simulink model "cukModelStateSpaceWithcontrol"  (R2020a)
settings: Solver=VariableStepAuto  StartTime=0.0  StopTime=0.3  RelTol=1e-9  AbsTol=4e-3
undefined symbols (not defined in the file): Asigma, b1, b2, bsigma, Csigma, Cxe, delta, f_s, fbounds, jthVec, Masigma, Mbsigma, Mcsigma, Nasigma, Nbsigma, Ncsigma, obsControl, obsSys, P, t_f, taua1, taua2, Tmax, uncertFreq, uncertType, x0, x_e, xe, xfdio0, xhat0
libraries: PhdLibrary x23, dspsigops x7, powerlib_meascontrol x5, dspmathops x1
(part 1 of 2)
settings Model: SimulationMode=accelerator  Creator=d13go  LastModifiedBy=d13go
settings SolverCC: ZeroCrossControl=DisableAll  ZeroCrossAlgorithm=Adaptive
settings DebuggingCC: IgnoredZcDiagnostic=none

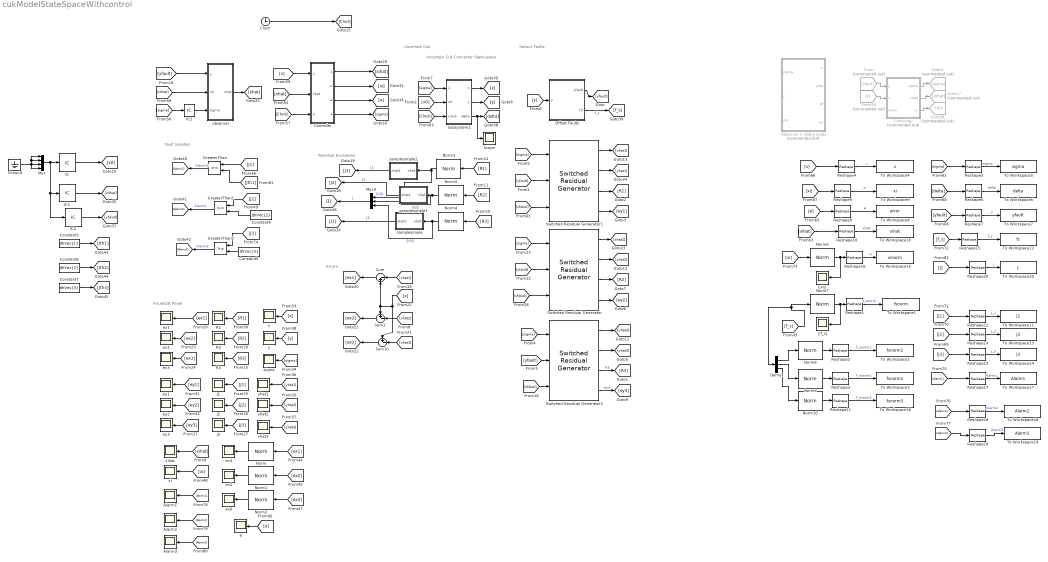
== system cukModelStateSpaceWithcontrol ==
  note: Errors
  note: Fault Isolation
  note: Visualizat Panel
  note: Sensor Faults
  note: Uncertain Cuk Converter
      | State-space
  note: Uncertain Cuk
  note: Residual Evaluation
  Alarm1 : Scope
  Alarm2 : Scope
  Alarm3 : Scope
  Clock : Clock
  Constant3 : Constant  Value=jthVec{1}
  Constant4 : Constant  Value=jthVec{2}
  Constant5 : Constant  Value=jthVec{3}
  Constant6 : Constant  Value=jthVec{2}
  Constant7 : Constant  Value=jthVec{3}
  Controler : Subsystem
  Controller : Subsystem  Commented=on
  Demux : Demux  Outputs=3
  From : From  Commented=on  GotoTag=yfault
  From50 : From  Commented=on  GotoTag=x
  Goto17 : Goto  Commented=on  GotoTag=xihat
  Goto28 : Goto  Commented=on  GotoTag=xi
  Goto4 : Goto  Commented=on  GotoTag=sigma
  GreaterThan : RelationalOperator  OutDataTypeStr=boolean  RndMeth=Simplest
  GreaterThan1 : RelationalOperator  OutDataTypeStr=boolean  RndMeth=Simplest
  GreaterThan2 : RelationalOperator  OutDataTypeStr=boolean  RndMeth=Simplest
  Ground : Ground
  IC : InitialCondition  Value=[x0]
  IC1 : InitialCondition  Value=[xhat0]
  IC2 : InitialCondition  Value=2
  IC4 : InitialCondition  Value=[xfdio0]
  J1 : Scope
  J2 : Scope
  J3 : Scope
  Mux : Mux
  Mux4 : Mux  Inputs=3
  Norm{,1..10} (11 alike) : PhdLibrary/Norms/Norm
      settings: SourceProductName=Phd Diego
  Observer 2 slidng mode : Subsystem  Commented=on  mask(Boots State-Space model){A1=obsSys{3}.Asigma{1,1}, A2=obsSys{3}.Asigma{1,2}, B1=obsSys{3}.bsigma{1,1}, Cmatrix=obsSys{3}.Csigma{1,1}, L1=obsSys{3}.Lsigma{1,1}, L2=obsSys{3}.Lsigma{1,2}, Gn1=obsSys{3}.Gnsigma{1,1}, Gn2=obsSys{3}.Gnsigma{1,2}, Po=obsSys{3}.Po, R1=obsSys{3}.Rsigma{1,1}, R2=obsSys{3}.Rsigma{1,2}, delta=delta}
      mask prompts: A1 "A1 matrix"; A2 "A2 matrix"; B1 "B matrix"; Cmatrix "Output Matrix"; L1 "L1 matrix"; L2 "L2 matrix"; Gn1 "Gn1 matrix"; Gn2 "Gn2 matrix"; Po "Po matrix"; R1 "R1 matrix"; R2 "R2 matrix"; delta "Delta Sliding mode"
      mask help: Boots State-Space model
      mask Display: disp('Observer')
  Offset Faults : Subsystem
  R1 : Scope
  R2 : Scope
  R3 : Scope
  Reshape{1..20} (20 alike) : Reshape
  Scope : Scope
  Subsystem2 : Subsystem
  Sum : Sum  Inputs=|-+
  Sum1 : Sum  Inputs=+-|
  Sum10 : Sum  Inputs=+-|
  Switched Residual Generator : PhdLibrary/Observers/Switched Residual Generator  A1=obsSys{2}.Asigma{1,1}  B1=obsSys{2}.bsigma{1,1}  L1=obsSys{2}.Lsigma{1,1}  C1=obsSys{2}.Csigma{1,1}  R1=obsSys{2}.Rsigma{1,1}  A2=obsSys{2}.Asigma{1,2}  B2=obsSys{2}.bsigma{1,1}  C2=obsSys{2}.Csigma{1,1}  L2=obsSys{2}.Lsigma{1,2}  R2=obsSys{2}.Rsigma{1,2}
      settings: SourceProductName=Phd Diego
  Switched Residual Generator1 : PhdLibrary/Observers/Switched Residual Generator  A1=obsSys{1}.Asigma{1,1}  B1=obsSys{1}.bsigma{1,1}  L1=obsSys{1}.Lsigma{1,1}  C1=obsSys{1}.Csigma{1,1}  R1=obsSys{1}.Rsigma{1,1}  A2=obsSys{1}.Asigma{1,2}  B2=obsSys{1}.bsigma{1,1}  C2=obsSys{1}.Csigma{1,1}  L2=obsSys{1}.Lsigma{1,2}  R2=obsSys{1}.Rsigma{1,2}
      settings: SourceProductName=Phd Diego
  Switched Residual Generator2 : PhdLibrary/Observers/Switched Residual Generator  A1=obsSys{3}.Asigma{1,1}  B1=obsSys{3}.bsigma{1,1}  L1=obsSys{3}.Lsigma{1,1}  C1=obsSys{3}.Csigma{1,1}  R1=obsSys{3}.Rsigma{1,1}  A2=obsSys{3}.Asigma{1,2}  B2=obsSys{3}.bsigma{1,1}  C2=obsSys{3}.Csigma{1,1}  L2=obsSys{3}.Lsigma{1,2}  R2=obsSys{3}.Rsigma{1,2}
      settings: SourceProductName=Phd Diego
  To Workspace1 : ToWorkspace  VariableName=fsnorm  SaveFormat=Timeseries  SampleTime=-1
  To Workspace10 : ToWorkspace  VariableName=xihat  SaveFormat=Timeseries  SampleTime=-1
  To Workspace11 : ToWorkspace  VariableName=J1  SaveFormat=Timeseries  SampleTime=-1
  To Workspace12 : ToWorkspace  VariableName=fs  SaveFormat=Timeseries  SampleTime=-1
  To Workspace13 : ToWorkspace  VariableName=J2  SaveFormat=Timeseries  SampleTime=-1
  To Workspace14 : ToWorkspace  VariableName=J3  SaveFormat=Timeseries  SampleTime=-1
  To Workspace15 : ToWorkspace  VariableName=xinorm  SaveFormat=Timeseries  SampleTime=-1
  To Workspace16 : ToWorkspace  VariableName=fsnorm3  SaveFormat=Timeseries  SampleTime=-1
  To Workspace17 : ToWorkspace  VariableName=Alarm1  SaveFormat=Timeseries  SampleTime=-1
  To Workspace18 : ToWorkspace  VariableName=Alarm2  SaveFormat=Timeseries  SampleTime=-1
  To Workspace19 : ToWorkspace  VariableName=Alarm3  SaveFormat=Timeseries  SampleTime=-1
  To Workspace2 : ToWorkspace  VariableName=fsnorm1  SaveFormat=Timeseries  SampleTime=-1
  To Workspace20 : ToWorkspace  VariableName=J  SaveFormat=Timeseries  SampleTime=-1
  To Workspace3 : ToWorkspace  VariableName=fsnorm2  SaveFormat=Timeseries  SampleTime=-1
  To Workspace4 : ToWorkspace  VariableName=x  SaveFormat=Timeseries  SampleTime=-1
  To Workspace5 : ToWorkspace  VariableName=sigma  SaveFormat=Timeseries  SampleTime=-1
  To Workspace6 : ToWorkspace  VariableName=delta  SaveFormat=Timeseries  SampleTime=-1
  To Workspace7 : ToWorkspace  VariableName=yfault  SaveFormat=Timeseries  SampleTime=-1
  To Workspace8 : ToWorkspace  VariableName=error  SaveFormat=Timeseries  SampleTime=-1
  To Workspace9 : ToWorkspace  VariableName=xi  SaveFormat=Timeseries  SampleTime=-1
  e : Scope
  ex{1..6} (6 alike) : Scope
  ey1 : Scope
  ey2 : Scope
  ey3 : Scope
  observer : Subsystem
  samplesimple : Subsystem
  samplesimple1 : Subsystem
  samplesimple2 : Subsystem
  sigma : Scope
  x : Scope
  xi : Scope
  xihat : Scope
  y : Scope
  yhat1 : Scope
  yhat2 : Scope
  yhat3 : Scope
  ||f_s| : Scope
  ||xi|| : Scope
  wires:
  Subsystem2/1(x) -> [x]
  Clock/1 -> [Clock]
  [sigma] -> Switched Residual Generator1/1
  Switched Residual Generator1/3 -> [R1]
  [sigma] -> Switched Residual Generator/1
  [yfault] -> Switched Residual Generator/2
  Switched Residual Generator1/4 -> [ey1]
  [yfault] -> Switched Residual Generator2/2
  [sigma] -> Switched Residual Generator2/1
  Switched Residual Generator2/2 -> [yhat3]
  Subsystem2/2(y) -> [y]
  Switched Residual Generator2/1 -> [xhat3]
  [xhat3] -> Sum10/2
  [yfault] -> Switched Residual Generator1/2
  [y] -> Offset Faults/1(y)
  Offset Faults/1(yfault) -> [yfault]
  Controller/1(sigma) -> Goto4/1
  From/1 -> Controller/1(y)
  [sigma] -> Subsystem2/1(sigma)
  [xhat2] -> Sum1/2
  Mux/1 -> IC1/1, IC4/1, IC/1
  Switched Residual Generator2/4 -> [ey3]  "ey3"
  Switched Residual Generator1/1 -> [xhat1]
  Switched Residual Generator2/3 -> [R3]  "R3"
  IC/1 -> [x0]
  [xfdio0] -> Switched Residual Generator2/3
  Ground/1 -> Mux/4, Mux/1, Mux/2, Mux/3
  [R3] -> Norm4/1
  Norm4/1 -> Mux4/3, samplesimple/1(xhat)  "||r3||"
  Norm5/1 -> samplesimple1/1(xhat), Mux4/2  "||r2||"
  [R2] -> Norm5/1
  Norm3/1 -> samplesimple2/1(xhat), Mux4/1  "||r1||"
  [R1] -> Norm3/1
  [R3] -> R3/1
  [ey3] -> ey3/1
  [xhat1] -> Sum/1
  [x] -> Sum/2, Sum1/1, Sum10/1
  Sum/1 -> [ex1]
  Sum10/1 -> [ex3]
  Sum1/1 -> [ex2]
  [ex1] -> ex1/1
  [ex2] -> ex2/1
  [ex3] -> ex3/1
  [J1] -> J1/1
  [J3] -> J3/1
  [J2] -> J2/1
  [xfdio0] -> Switched Residual Generator/3
  Switched Residual Generator/3 -> [R2]
  Switched Residual Generator/4 -> [ey2]
  Switched Residual Generator/2 -> [yhat2]
  Switched Residual Generator/1 -> [xhat2]
  [xfdio0] -> Switched Residual Generator1/3
  Switched Residual Generator1/2 -> [yhat1]
  [R2] -> R2/1
  [R1] -> R1/1
  [ey1] -> ey1/1
  [ey2] -> ey2/1
  [x] -> x/1
  [sigma] -> sigma/1
  [yhat2] -> yhat2/1
  [yhat1] -> yhat1/1
  [yhat3] -> yhat3/1
  [y] -> y/1
  [ex1] -> Norm/1
  Norm/1 -> ex4/1
  Norm1/1 -> ex5/1
  [ex2] -> Norm1/1
  Norm2/1 -> ex6/1
  [ex3] -> Norm2/1
  Controller/2(xihat) -> Goto17/1
  Controller/3(xi) -> Goto28/1
  [xihat] -> xihat/1
  [xi] -> xi/1
  From50/1 -> Controller/2(x)
  IC2/1 -> observer/3(sigma)
  [xhat] -> Controler/2(xhat)
  observer/1(xhat) -> [xhat]
  [x] -> Controler/1(x)
  [sigma] -> IC2/1
  [Clock] -> Controler/3(clock)
  Controler/4(sigma) -> [sigma]
  Controler/3(e) -> [e]
  Controler/2(xi) -> [xi]
  Controler/1(xihat) -> [xihat]
  [yfault] -> observer/1(y)
  [x0hat] -> observer/2(x0)
  IC1/1 -> [x0hat]
  [e] -> e/1
  IC4/1 -> [xfdio0]
  [x0] -> Subsystem2/2(x0)
  [e] -> Reshape8/1
  Reshape4/1 -> To Workspace4/1  "x"
  Reshape8/1 -> To Workspace8/1  "e"
  [delta] -> Reshape6/1
  Reshape5/1 -> To Workspace5/1  "sigma"
  Reshape7/1 -> To Workspace7/1  "y"
  Reshape6/1 -> To Workspace6/1  "delta"
  [yfault] -> Reshape7/1
  [sigma] -> Reshape5/1
  [x] -> Reshape4/1
  [xi] -> Reshape9/1
  Reshape9/1 -> To Workspace9/1  "xi"
  Reshape10/1 -> To Workspace10/1  "xihat"
  [xihat] -> Reshape10/1
  Reshape12/1 -> To Workspace11/1  "J_1"
  [J1] -> Reshape12/1
  Reshape13/1 -> To Workspace14/1  "J_3"
  Reshape14/1 -> To Workspace13/1  "J_2"
  [J2] -> Reshape14/1
  [J3] -> Reshape13/1
  Offset Faults/2(f3) -> [f_s]  "f_s"
  Reshape15/1 -> To Workspace12/1  "f_s"
  [f_s] -> Reshape15/1
  Reshape16/1 -> To Workspace15/1  "xi"
  [xi] -> Norm6/1
  Norm6/1 -> ||xi||/1, Reshape16/1
  Norm7/1 -> ||f_s|/1, Reshape1/1
  Reshape1/1 -> To Workspace1/1  "f_snorm"
  [f_s] -> Norm7/1, Demux/1
  Reshape2/1 -> To Workspace2/1  "f_snorm1"
  Demux/1 -> Norm8/1
  Norm8/1 -> Reshape2/1
  Norm9/1 -> Reshape3/1
  Reshape3/1 -> To Workspace3/1  "f_snorm2"
  Demux/2 -> Norm9/1
  Reshape11/1 -> To Workspace16/1  "f_snorm3"
  Demux/3 -> Norm10/1
  Norm10/1 -> Reshape11/1
  [J1] -> GreaterThan/1
  [Jth1] -> GreaterThan/2
  Constant5/1 -> GreaterThan2/2
  [J3] -> GreaterThan2/1
  [J2] -> GreaterThan1/1
  Constant4/1 -> GreaterThan1/2
  GreaterThan/1 -> [Alarm1]  "Alarrm1"
  GreaterThan2/1 -> [Alarm3]  "Alarm3"
  GreaterThan1/1 -> [Alarm2]  "Alarm2"
  Reshape17/1 -> To Workspace17/1  "Alarm1"
  [Alarm1] -> Reshape17/1
  [Alarm2] -> Reshape18/1
  Reshape18/1 -> To Workspace18/1  "Alarm2"
  [Alarm3] -> Reshape19/1
  Reshape19/1 -> To Workspace19/1  "Alarm3"
  [Alarm1] -> Alarm1/1
  [Alarm2] -> Alarm2/1
  [Alarm3] -> Alarm3/1
  Constant3/1 -> [Jth1]
  Constant6/1 -> [Jth2]
  Constant7/1 -> [Jth3]
  Reshape20/1 -> To Workspace20/1  "J"
  [J] -> Reshape20/1
  [Clock] -> Subsystem2/3(clock)
  samplesimple1/1("xhatk ") -> [J2]  "J2"
  samplesimple2/1("xhatk ") -> [J1]  "J1"
  Mux4/1 -> [J]  "J"
  samplesimple/1("xhatk ") -> [J3]  "J3"
  Subsystem2/3(delta) -> Scope/1, [delta]

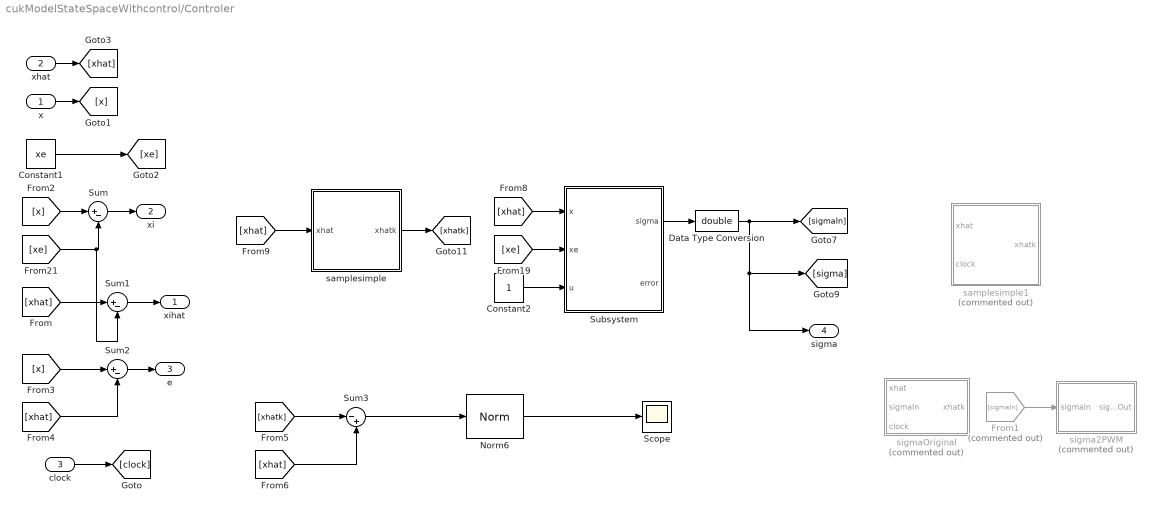
== system cukModelStateSpaceWithcontrol/Controler ==
  x : Inport
  xhat : Inport  Port=2
  clock : Inport  Port=3
  Constant1 : Constant  Value=xe  VectorParams1D=off
  Constant2 : Constant
  Data Type Conversion : DataTypeConversion  OutDataTypeStr=double
  From1 : From  Commented=on  GotoTag=sigmaIn
  Norm6 : PhdLibrary/Norms/Norm
      settings: SourceProductName=Phd Diego
  Scope : Scope
  Subsystem : Subsystem  mask{P1=P, A1=obsControl.Asigma{1}, B1=obsControl.bsigma{1}, P2=P, A2=obsControl.Asigma{2}, B2=obsControl.bsigma{2}}
      mask prompts: P1 "P matrx"; A1 "A matrix"; B1 "b matrix"; P2 "P matrx"; A2 "A matrix"; B2 "b matrix"
      mask DialogControl Container3 Prompt: Subsystem 1
      mask DialogControl Container3_copy Prompt: Subsystem 2
      mask Display: disp('Switching \n Control Law \n 2-Subsystems');
  Sum : Sum  Inputs=|+-
  Sum1 : Sum  Inputs=|+-
  Sum2 : Sum  Inputs=|+-
  Sum3 : Sum  Inputs=|-+
  samplesimple : Subsystem
  samplesimple1 : Subsystem  Commented=on
  sigma2PWM : Subsystem  Commented=on
  sigmaOriginal : Subsystem  Commented=on
  xihat : Outport
  xi : Outport  Port=2
  e : Outport  Port=3
  sigma : Outport  Port=4
  wires:
  [xe] -> Sum1/2, Sum/2
  xhat/1 -> [xhat]
  x/1 -> [x]
  Sum2/1 -> e/1
  samplesimple/1("xhatk ") -> [xhatk]
  Sum1/1 -> xihat/1
  [xe] -> Subsystem/2(xe)
  Constant2/1 -> Subsystem/3(u)
  Subsystem/1(sigma) -> Data Type Conversion/1
  Data Type Conversion/1 -> sigma/1, [sigma], [sigmaIn]
  From1/1 -> sigma2PWM/1(sigmaIn)
  clock/1 -> [clock]
  Sum/1 -> xi/1
  Constant1/1 -> [xe]
  [xhat] -> Sum1/1
  [x] -> Sum/1
  [x] -> Sum2/1
  [xhat] -> Sum2/2
  [xhatk] -> Sum3/1
  Sum3/1 -> Norm6/1
  [xhat] -> Sum3/2
  Norm6/1 -> Scope/1
  [xhat] -> samplesimple/1(xhat)
  [xhat] -> Subsystem/1(x)

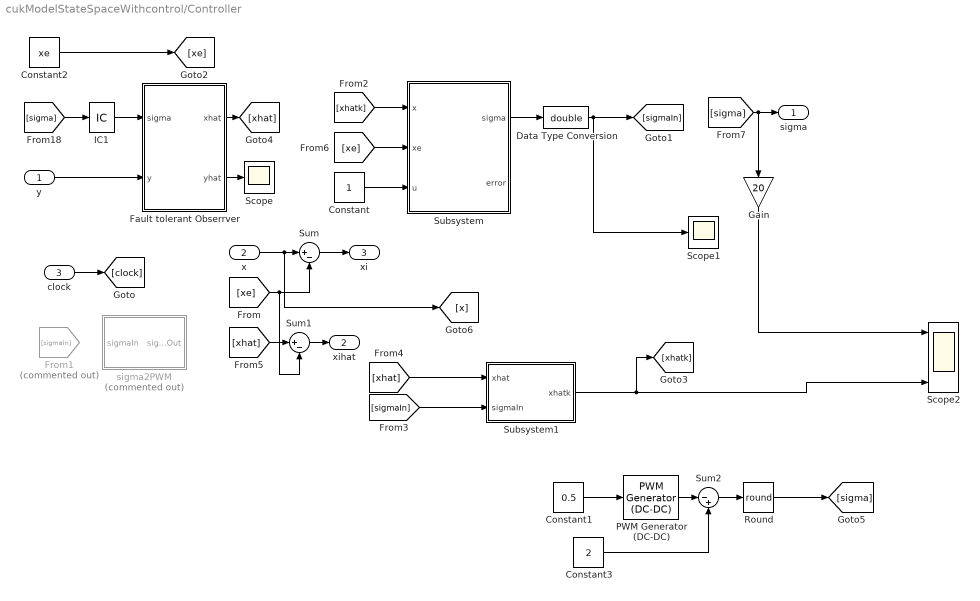
== system cukModelStateSpaceWithcontrol/Controller ==
  y : Inport
  x : Inport  Port=2
  clock : Inport  Port=3
  Constant : Constant
  Constant1 : Constant  Value=0.5
  Constant2 : Constant  Value=xe  VectorParams1D=off
  Constant3 : Constant  Value=2
  Data Type Conversion : DataTypeConversion  OutDataTypeStr=double
  Fault tolerant Obserrver : Subsystem  mask(Boots State-Space model){A1=obsControl.Asigma{1,1}, A2=obsControl.Asigma{1,2}, B1=obsControl.bsigma{1,1}, Cmatrix=obsControl.Csigma{1,1}, L1=obsControl.Lcsigma{1,1}, L2=obsControl.Lcsigma{1,2}}
      mask prompts: A1 "A1 matrix"; A2 "A2 matrix"; B1 "B matrix"; Cmatrix "Output Matrix"; L1 "L1 matrix"; L2 "L2 matrix"
      mask help: Boots State-Space model
      mask Display: disp('Observer')
  From1 : From  Commented=on  GotoTag=sigmaIn
  Gain : Gain  Gain=20
  IC1 : InitialCondition  Value=2
  PWM Generator (DC-DC) : powerlib_meascontrol/Pulse & Signal Generators/PWM Generator (DC-DC)  Fsw=10000  Ts=5e-6
  Round : Rounding  Operator=round
  Scope : Scope
  Scope1 : Scope
  Scope2 : Scope  NumInputPorts=3
  Subsystem : Subsystem  mask{P1=obsControl.P{1}, A1=obsControl.Asigma{1}, B1=obsControl.bsigma{1}, P2=obsControl.P{2}, A2=obsControl.Asigma{2}, B2=obsControl.bsigma{2}}
      mask prompts: P1 "P matrx"; A1 "A matrix"; B1 "b matrix"; P2 "P matrx"; A2 "A matrix"; B2 "b matrix"
      mask DialogControl Container3 Prompt: Subsystem 1
      mask DialogControl Container3_copy Prompt: Subsystem 2
      mask Display: disp('Switching \n Control Law \n 2-Subsystems');
  Subsystem1 : Subsystem
  Sum : Sum  Inputs=|+-
  Sum1 : Sum  Inputs=|+-
  Sum2 : Sum  Inputs=|-+
  sigma2PWM : Subsystem  Commented=on
  sigma : Outport
  xihat : Outport  Port=2
  xi : Outport  Port=3
  wires:
  [sigma] -> IC1/1
  Fault tolerant Obserrver/2(yhat) -> Scope/1
  y/1 -> Fault tolerant Obserrver/2(y)
  Fault tolerant Obserrver/1(xhat) -> [xhat]
  Constant2/1 -> [xe]
  IC1/1 -> Fault tolerant Obserrver/1(sigma)
  Constant/1 -> Subsystem/3(u)
  x/1 -> [x], Sum/1
  [xe] -> Sum/2, Sum1/2
  Sum/1 -> xi/1
  clock/1 -> [clock]
  Subsystem/1(sigma) -> Data Type Conversion/1
  Data Type Conversion/1 -> Scope1/1, [sigmaIn]
  [sigma] -> Gain/1, sigma/1
  Gain/1 -> Scope2/1
  Subsystem1/1("xhatk ") -> [xhatk], Scope2/3
  [sigmaIn] -> Subsystem1/2(sigmaIn)
  [xhat] -> Sum1/1
  Sum1/1 -> xihat/1
  [xe] -> Subsystem/2(xe)
  [xhat] -> Subsystem1/1(xhat)
  [xhatk] -> Subsystem/1(x)
  Constant1/1 -> PWM Generator (DC-DC)/1
  Constant3/1 -> Sum2/2
  Sum2/1 -> Round/1
  PWM Generator (DC-DC)/1 -> Sum2/1
  Round/1 -> [sigma]

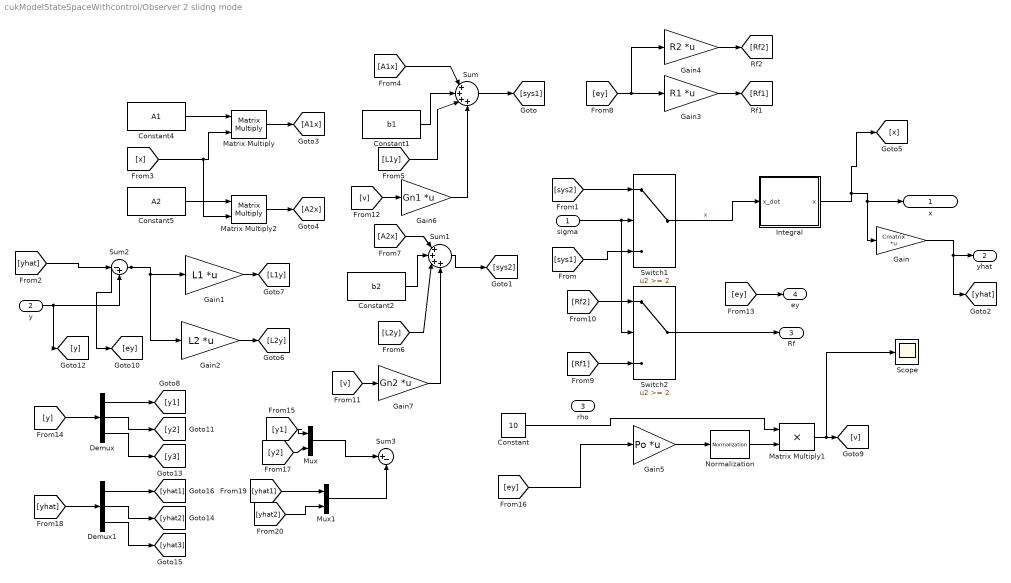
== system cukModelStateSpaceWithcontrol/Observer 2 slidng mode ==
  sigma : Inport
  y : Inport  Port=2
  rho : Inport  Port=3
  Constant : Constant  Value=10
  Constant1 : Constant  Value=b1  VectorParams1D=off
  Constant2 : Constant  Value=b2  VectorParams1D=off
  Constant4 : Constant  Value=A1  VectorParams1D=off
  Constant5 : Constant  Value=A2  VectorParams1D=off
  Demux : Demux  Outputs=3
  Demux1 : Demux  Outputs=3
  Gain : Gain  Gain=Cmatrix  Multiplication=Matrix(K*u)
  Gain1 : Gain  Gain=L1  Multiplication=Matrix(K*u) (u vector)
  Gain2 : Gain  Gain=L2  Multiplication=Matrix(K*u) (u vector)
  Gain3 : Gain  Gain=R1  Multiplication=Matrix(K*u) (u vector)
  Gain4 : Gain  Gain=R2  Multiplication=Matrix(K*u) (u vector)
  Gain5 : Gain  Gain=Po  Multiplication=Matrix(K*u) (u vector)
  Gain6 : Gain  Gain=Gn1  Multiplication=Matrix(K*u) (u vector)
  Gain7 : Gain  Gain=Gn2  Multiplication=Matrix(K*u) (u vector)
  Integral : Subsystem
  Matrix Multiply : Product  Multiplication=Matrix(*)
  Matrix Multiply1 : Product
  Matrix Multiply2 : Product  Multiplication=Matrix(*)
  Mux : Mux  Inputs=2
  Mux1 : Mux  Inputs=2
  Normalization : dspmathops/Normalization  NormType=2-norm  Bias=delta  NormOver=Each column  Dimension=1  roundingMode=Floor  overflowMode=off  accumDataTypeStr=Inherit: Same as product output  accumLastDataTypeStr=Inherit: Same as product output  outputDataTypeStr=Inherit: Same as product output  outputMin=[]  outputMax=[]  outputLastDataTypeStr=Inherit: Same as product output
  Scope : Scope
  Sum : Sum  Inputs=|++++
  Sum1 : Sum  Inputs=|++++
  Sum2 : Sum  Inputs=|-+
  Sum3 : Sum  Inputs=|+-
  Switch1 : Switch  Threshold=2
  Switch2 : Switch  Threshold=2
  x : Outport
  yhat : Outport  Port=2
  Rf : Outport  Port=3
  ey : Outport  Port=4
  wires:
  Gain/1 -> [yhat], yhat/1
  Constant1/1 -> Sum/2
  sigma/1 -> Switch2/2, Switch1/2
  Matrix Multiply2/1 -> [A2x]
  Sum/1 -> [sys1]
  Constant4/1 -> Matrix Multiply/1
  Constant2/1 -> Sum1/2
  Integral/1(x) -> [x], x/1, Gain/1
  Constant5/1 -> Matrix Multiply2/1
  [x] -> Matrix Multiply2/2, Matrix Multiply/2
  Matrix Multiply/1 -> [A1x]
  Sum1/1 -> [sys2]
  [A2x] -> Sum1/1
  [A1x] -> Sum/1
  [L2y] -> Sum1/3
  [yhat] -> Sum2/1
  y/1 -> [y], Sum2/2
  Sum2/1 -> Gain2/1, Gain1/1, [ey]
  Gain2/1 -> [L2y]
  Gain1/1 -> [L1y]
  [L1y] -> Sum/3
  [ey] -> Gain4/1, Gain3/1
  [sys2] -> Switch1/1
  [sys1] -> Switch1/3
  Gain3/1 -> [Rf1]
  Gain4/1 -> [Rf2]
  Switch1/1 -> Integral/1(x_dot)  "x"
  Switch2/1 -> Rf/1
  Gain5/1 -> Normalization/1
  Normalization/1 -> Matrix Multiply1/2
  [v] -> Gain6/1
  [ey] -> ey/1
  Matrix Multiply1/1 -> Scope/1, [v]
  [y] -> Demux/1
  Demux/1 -> [y1]
  Demux/2 -> [y2]
  Demux/3 -> [y3]
  [y1] -> Mux/1
  [y2] -> Mux/2
  [yhat] -> Demux1/1
  Demux1/2 -> [yhat2]
  Demux1/1 -> [yhat1]
  Demux1/3 -> [yhat3]
  [yhat1] -> Mux1/1
  [yhat2] -> Mux1/2
  Mux/1 -> Sum3/1
  Mux1/1 -> Sum3/2
  Constant/1 -> Matrix Multiply1/1
  [v] -> Gain7/1
  Gain7/1 -> Sum1/4
  Gain6/1 -> Sum/4
  [ey] -> Gain5/1
  [Rf1] -> Switch2/3
  [Rf2] -> Switch2/1

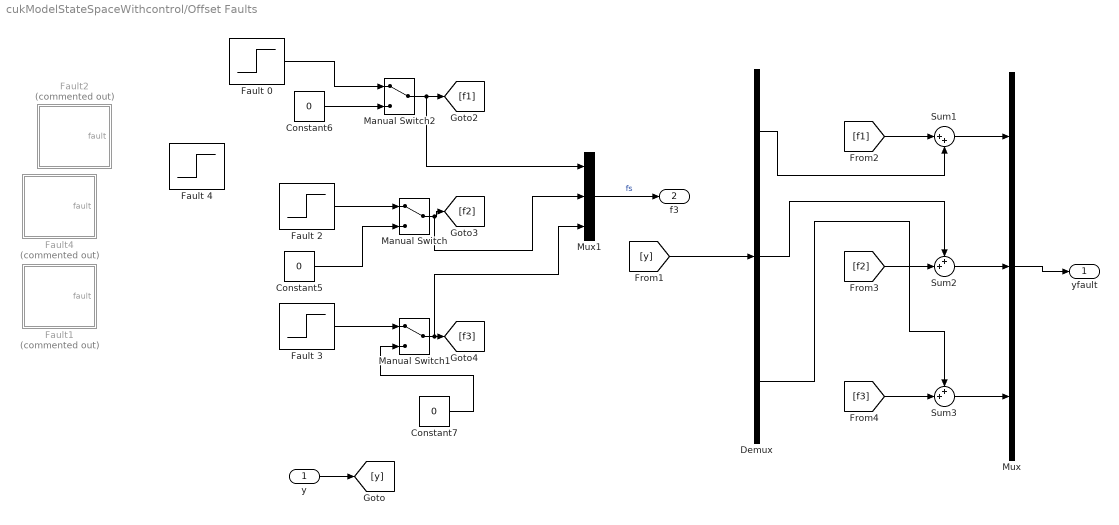
== system cukModelStateSpaceWithcontrol/Offset Faults ==
  y : Inport
  Constant5 : Constant  Value=0
  Constant6 : Constant  Value=0
  Constant7 : Constant  Value=0
  Demux : Demux  Outputs=3
  Fault 0 : Step  Time=t_f(1)  After=f_s(1)  SampleTime=0
  Fault 2 : Step  Time=t_f(2)  After=f_s(2)  SampleTime=0
  Fault 3 : Step  Time=t_f(3)  After=f_s(3)  SampleTime=0
  Fault 4 : Step  Time=t_f(3)  After=0.15*Cxe(3)  SampleTime=0
  Fault1 : Subsystem  Commented=on  mask{fbound=fbounds(1), t_f=t_f(1), f_freq_Hz=60}
      mask prompts: fbound "Maximum Bound"; t_f "Fault Time"; f_freq_Hz "Fault Frequency"
      mask Display: fprintf('Sinusoidal\nFault\nFunction')
  Fault2 : Subsystem  Commented=on  mask{fbound=fbounds(3), t_f=t_f(3), f_freq_Hz=60}
      mask prompts: fbound "Maximum Bound"; t_f "Fault Time"; f_freq_Hz "Fault Frequency"
      mask Display: fprintf('Sinusoidal\nFault\nFunction')
  Fault4 : Subsystem  Commented=on  mask{fbound=fbounds(2), t_f=t_f(2), f_freq_Hz=60}
      mask prompts: fbound "Maximum Bound"; t_f "Fault Time"; f_freq_Hz "Fault Frequency"
      mask Display: fprintf('Sinusoidal\nFault\nFunction')
  Manual Switch : ManualSwitch
  Manual Switch1 : ManualSwitch
  Manual Switch2 : ManualSwitch
  Mux : Mux  Inputs=3
  Mux1 : Mux  Inputs=3
  Sum1 : Sum  Inputs=|++
  Sum2 : Sum  Inputs=++|
  Sum3 : Sum  Inputs=++|
  yfault : Outport
  f3 : Outport  Port=2
  wires:
  Mux/1 -> yfault/1
  Manual Switch1/1 -> Mux1/3, [f3]
  Constant5/1 -> Manual Switch/2
  Sum1/1 -> Mux/1
  Sum3/1 -> Mux/3
  y/1 -> [y]
  Sum2/1 -> Mux/2
  Manual Switch2/1 -> Mux1/1, [f1]
  [f1] -> Sum1/1
  Manual Switch/1 -> Mux1/2, [f2]
  [f2] -> Sum2/2
  [f3] -> Sum3/2
  [y] -> Demux/1
  Demux/1 -> Sum1/2
  Demux/2 -> Sum2/1
  Demux/3 -> Sum3/1
  Mux1/1 -> f3/1  "fs"
  Constant7/1 -> Manual Switch1/2
  Constant6/1 -> Manual Switch2/2
  Fault 3/1 -> Manual Switch1/1
  Fault 2/1 -> Manual Switch/1
  Fault 0/1 -> Manual Switch2/1

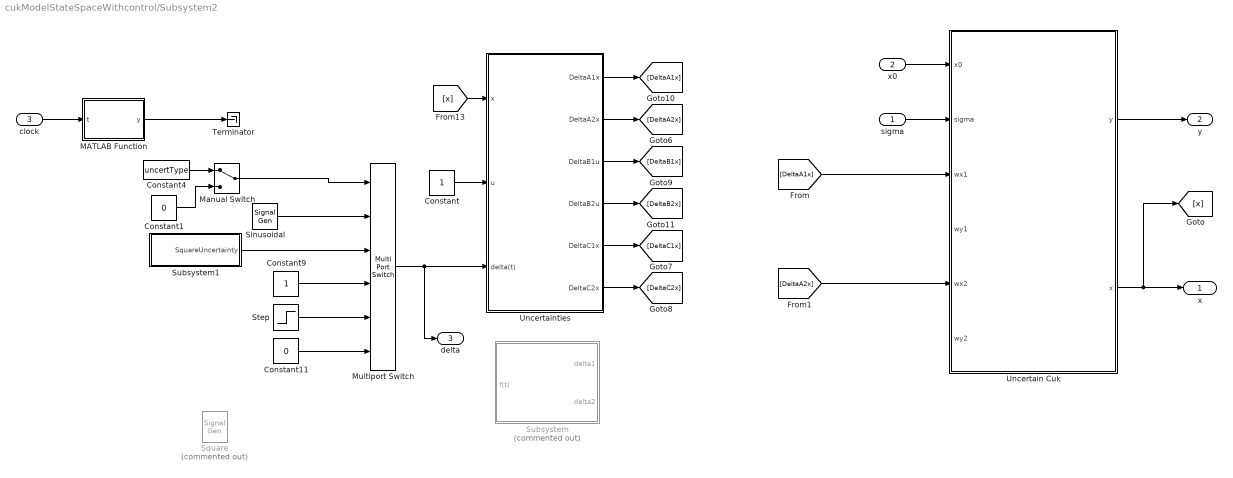
== system cukModelStateSpaceWithcontrol/Subsystem2 ==
  sigma : Inport
  x0 : Inport  Port=2
  clock : Inport  Port=3
  Constant : Constant
  Constant1 : Constant  Value=0
  Constant11 : Constant  Value=0
  Constant4 : Constant  Value=uncertType
  Constant9 : Constant
  MATLAB Function : MATLAB Function  TreatAsAtomicUnit=on
  Manual Switch : ManualSwitch
  Multiport Switch : MultiPortSwitch  Inputs=5
  Sinusoidal : SignalGenerator  Frequency=60  Units=rad/sec
  Square : SignalGenerator  Commented=on  WaveForm=square  Frequency=uncertFreq  Units=rad/sec
  Step : Step  Time=0.35  SampleTime=0
  Subsystem : Subsystem  Commented=on  mask{M1=Mbsigma{1,1}, M2=Mbsigma{1,2}, N1=Nbsigma{1,1}, N2=Nbsigma{1,2}}
      mask prompts: M1 "M matrix 1"; M2 "M matrix 2"; N1 "N matrix 1"; N2 "N matrix 2"
      mask DialogControl DescTextVar Prompt: Uncertainties matrices
      mask Display: disp('Norm-bounded \n uncertainty - Switched')
  Subsystem1 : Subsystem
  Terminator : Terminator
  Uncertain Cuk : Subsystem  mask{A1=Asigma{1}, B1=bsigma{1}, C1=Csigma{1}, A2=Asigma{2}, B2=bsigma{2}, C2=Csigma{2}}
      mask prompts: A1 "Matrix A"; B1 "Matrix B"; C1 "Matrix C"; A2 "Matrix A"; B2 "Matrix B"; C2 "Matrix C"
      mask DialogControl DescTextVar Prompt: dx/dt = A(sigma)x+ B(sigma)u + wx(sigma,x,u,t)
      mask DialogControl Control2 Prompt: y = C(sigma)x + wy(sigma,x,u,t)
      mask DialogControl Container3 Prompt: Subsystem 1
      mask DialogControl Container4 Prompt: Subsystem 2
      mask Display: disp('Switched Perturbed State Space \n 2-Subsystems')
  Uncertainties : Subsystem
  x : Outport
  y : Outport  Port=2
  delta : Outport  Port=3
  wires:
  Uncertainties/2(DeltaA2x) -> [DeltaA2x]
  Uncertain Cuk/2(x) -> [x], x/1
  Constant/1 -> Uncertainties/2(u)
  Uncertainties/4(DeltaB2u) -> [DeltaB2x]
  Uncertainties/1(DeltaA1x) -> [DeltaA1x]
  Uncertain Cuk/1(y) -> y/1
  sigma/1 -> Uncertain Cuk/2(sigma)
  Uncertainties/6(DeltaC2x) -> [DeltaC2x]
  [x] -> Uncertainties/1(x)
  Uncertainties/5(DeltaC1x) -> [DeltaC1x]
  Uncertainties/3(DeltaB1u) -> [DeltaB1x]
  [DeltaA1x] -> Uncertain Cuk/3(wx1)
  Constant9/1 -> Multiport Switch/4
  Multiport Switch/1 -> delta/1, Uncertainties/3(delta(t))
  Constant11/1 -> Multiport Switch/6
  Step/1 -> Multiport Switch/5
  x0/1 -> Uncertain Cuk/1(x0)
  Constant4/1 -> Manual Switch/1
  Manual Switch/1 -> Multiport Switch/1
  Constant1/1 -> Manual Switch/2
  clock/1 -> MATLAB Function/1(t)
  Sinusoidal/1 -> Multiport Switch/2
  MATLAB Function/1(y) -> Terminator/1
  [DeltaA2x] -> Uncertain Cuk/5(wx2)
  Subsystem1/1(SquareUncertainty) -> Multiport Switch/3

== system cukModelStateSpaceWithcontrol/observer ==
  y : Inport
  x0 : Inport  Port=2
  sigma : Inport  Port=3
  Fault tolerant Obserrver : Subsystem  mask(Boots State-Space model){A1=obsControl.Asigma{1,1}, A2=obsControl.Asigma{1,2}, B1=obsControl.bsigma{1,1}, Cmatrix=obsControl.Csigma{1,1}, L1=obsControl.Lcsigma{1,1}, L2=obsControl.Lcsigma{1,2}}
      mask prompts: A1 "A1 matrix"; A2 "A2 matrix"; B1 "B matrix"; Cmatrix "Output Matrix"; L1 "L1 matrix"; L2 "L2 matrix"
      mask help: Boots State-Space model
      mask Display: disp('Observer')
  Terminator : Terminator
  xhat : Outport
  wires:
  y/1 -> Fault tolerant Obserrver/2(y)
  Fault tolerant Obserrver/1(xhat) -> xhat/1, [xhat]
  sigma/1 -> Fault tolerant Obserrver/1(sigma)
  x0/1 -> Fault tolerant Obserrver/3(x0)
  Fault tolerant Obserrver/2(yhat) -> Terminator/1

== system cukModelStateSpaceWithcontrol/samplesimple ==
  xhat : Inport
  NOT : Logic  Operator=NOT  IconShape=distinctive  AllPortsSameDT=off  OutDataTypeStr=boolean
  Pulse Generator : DiscretePulseGenerator  PulseType=Time based  Period=2*10e-6  PulseWidth=50
  Sample and Hold : dspsigops/Sample and Hold  trig=Either edge  initCond=0  latchinput=off
  Scope : Scope
  "xhatk " : Outport
  wires:
  xhat/1 -> Sample and Hold/1
  Sample and Hold/1 -> Scope/1, "xhatk "/1
  Pulse Generator/1 -> NOT/1
  NOT/1 -> Sample and Hold/Trigger

== system cukModelStateSpaceWithcontrol/samplesimple1 ==
  xhat : Inport
  NOT : Logic  Operator=NOT  IconShape=distinctive  AllPortsSameDT=off  OutDataTypeStr=boolean
  Pulse Generator : DiscretePulseGenerator  PulseType=Time based  Period=2*10e-6  PulseWidth=50
  Sample and Hold : dspsigops/Sample and Hold  trig=Either edge  initCond=0  latchinput=off
  Scope : Scope
  "xhatk " : Outport
  wires:
  xhat/1 -> Sample and Hold/1
  Sample and Hold/1 -> Scope/1, "xhatk "/1
  Pulse Generator/1 -> NOT/1
  NOT/1 -> Sample and Hold/Trigger

== system cukModelStateSpaceWithcontrol/samplesimple2 ==
  xhat : Inport
  NOT : Logic  Operator=NOT  IconShape=distinctive  AllPortsSameDT=off  OutDataTypeStr=boolean
  Pulse Generator : DiscretePulseGenerator  PulseType=Time based  Period=2*10e-6  PulseWidth=50
  Sample and Hold : dspsigops/Sample and Hold  trig=Either edge  initCond=0  latchinput=off
  Scope : Scope
  "xhatk " : Outport
  wires:
  xhat/1 -> Sample and Hold/1
  Sample and Hold/1 -> Scope/1, "xhatk "/1
  Pulse Generator/1 -> NOT/1
  NOT/1 -> Sample and Hold/Trigger

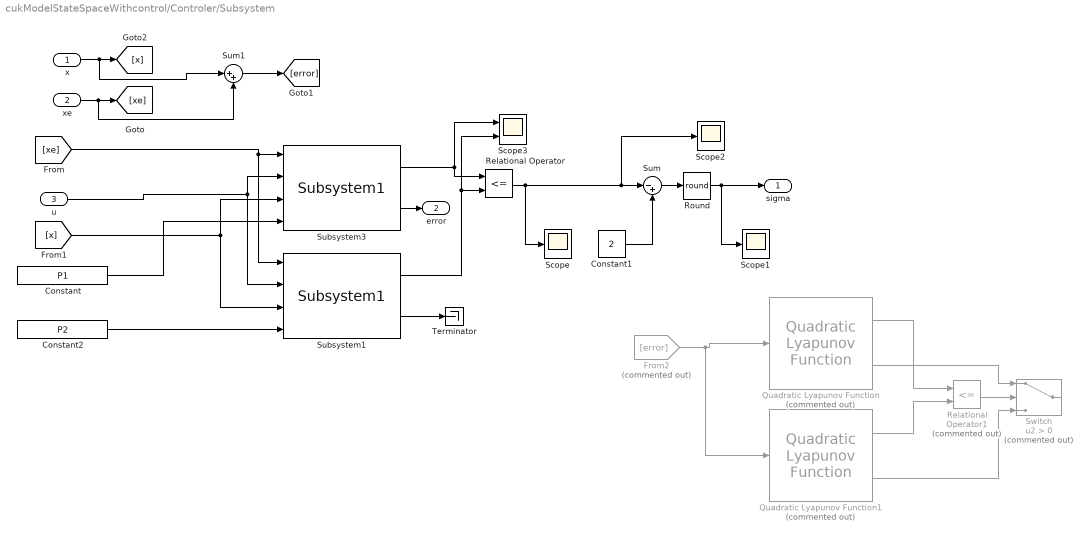
== system cukModelStateSpaceWithcontrol/Controler/Subsystem ==
  x : Inport
  xe : Inport  Port=2
  u : Inport  Port=3
  Constant : Constant  Value=P1
  Constant1 : Constant  Value=2
  Constant2 : Constant  Value=P2
  From2 : From  Commented=on  GotoTag=error
  Quadratic Lyapunov Function : PhdLibrary/Quadratic Lyapunov Function  Commented=on  P=P1
      settings: SourceProductName=Phd Diego
  Quadratic Lyapunov Function1 : PhdLibrary/Quadratic Lyapunov Function  Commented=on  P=P2
      settings: SourceProductName=Phd Diego
  Relational Operator : RelationalOperator  Operator=<=  OutDataTypeStr=boolean  RndMeth=Nearest
  Relational Operator1 : RelationalOperator  Commented=on  Operator=<=  OutDataTypeStr=boolean  RndMeth=Nearest
  Round : Rounding  Operator=round
  Scope : Scope
  Scope1 : Scope
  Scope2 : Scope
  Scope3 : Scope  NumInputPorts=2
  Subsystem1 : PhdLibrary/Controllers/Subsystem1  A=A2  B=B2
      settings: SourceProductName=Phd Diego
  Subsystem3 : PhdLibrary/Controllers/Subsystem1  A=A1  B=B1
      settings: SourceProductName=Phd Diego
  Sum : Sum  Inputs=|-+
  Sum1 : Sum  Inputs=|++
  Switch : Switch  Commented=on  Criteria=u2 > Threshold
  Terminator : Terminator
  sigma : Outport
  error : Outport  Port=2
  wires:
  x/1 -> Sum1/1, [x]
  [xe] -> Subsystem1/1, Subsystem3/1
  [x] -> Subsystem1/3, Subsystem3/3
  u/1 -> Subsystem1/2, Subsystem3/2
  Subsystem1/2 -> Terminator/1
  Subsystem3/2 -> error/1
  Subsystem1/1 -> Scope3/2, Relational Operator/2
  Subsystem3/1 -> Relational Operator/1, Scope3/1
  Relational Operator/1 -> Scope2/1, Sum/1, Scope/1
  Constant1/1 -> Sum/2
  Sum/1 -> Round/1
  Round/1 -> Scope1/1, sigma/1
  xe/1 -> [xe], Sum1/2
  Sum1/1 -> [error]
  From2/1 -> Quadratic Lyapunov Function1/1, Quadratic Lyapunov Function/1
  Quadratic Lyapunov Function1/1 -> Relational Operator1/2
  Relational Operator1/1 -> Switch/2
  Quadratic Lyapunov Function1/2 -> Switch/3
  Quadratic Lyapunov Function/1 -> Relational Operator1/1
  Quadratic Lyapunov Function/2 -> Switch/1
  Constant/1 -> Subsystem3/4
  Constant2/1 -> Subsystem1/4

== system cukModelStateSpaceWithcontrol/Controler/samplesimple ==
  xhat : Inport
  NOT : Logic  Operator=NOT  IconShape=distinctive  AllPortsSameDT=off  OutDataTypeStr=boolean
  Pulse Generator : DiscretePulseGenerator  PulseType=Time based  Period=2*10e-6  PulseWidth=50
  Sample and Hold : dspsigops/Sample and Hold  trig=Either edge  initCond=1  latchinput=off
  Scope : Scope
  "xhatk " : Outport
  wires:
  xhat/1 -> Sample and Hold/1
  Sample and Hold/1 -> Scope/1, "xhatk "/1
  Pulse Generator/1 -> NOT/1
  NOT/1 -> Sample and Hold/Trigger

== system cukModelStateSpaceWithcontrol/Controler/samplesimple1 ==
  xhat : Inport
  clock : Inport  Port=2
  Constant : Constant  Value=Tmax{1}
  GreaterThan : RelationalOperator  OutDataTypeStr=boolean  RndMeth=Simplest
  IC1 : InitialCondition  Value=0
  IC2 : InitialCondition  Value=0
  Memory1 : Memory  InheritSampleTime=on
  Memory2 : Memory  InheritSampleTime=on
  Sample and Hold : dspsigops/Sample and Hold  trig=Rising edge  initCond=1  latchinput=off
  Scope5 : Scope
  Sum : Sum  Inputs=|+-
  Switch2 : Switch  Criteria=u2 ~= 0
  "xhatk " : Outport
  wires:
  xhat/1 -> Sample and Hold/1
  Sample and Hold/1 -> "xhatk "/1
  [clock] -> Sum/1
  Sum/1 -> Scope5/1, [terror]
  Constant/1 -> GreaterThan/2
  [terror] -> GreaterThan/1
  GreaterThan/1 -> [reset], Sample and Hold/Trigger
  clock/1 -> [clock], Switch2/1
  [newclock] -> IC1/1
  IC1/1 -> Sum/2
  Switch2/1 -> [newclock], Memory2/1
  Memory2/1 -> Switch2/3
  [reset] -> IC2/1
  Memory1/1 -> Switch2/2
  IC2/1 -> Memory1/1

== system cukModelStateSpaceWithcontrol/Controler/sigma2PWM ==
  sigmaIn : Inport
  Constant1 : Constant
  Constant10 : Constant  Value=2
  Constant3 : Constant  Value=0
  PWM Generator (DC-DC) : powerlib_meascontrol/Pulse & Signal Generators/PWM Generator (DC-DC)  Fsw=1  Ts=5e-6
  Sum9 : Sum  Inputs=|-+
  Switch1 : Switch  Threshold=2
  sigmaOut : Outport
  wires:
  Switch1/1 -> PWM Generator (DC-DC)/1
  PWM Generator (DC-DC)/1 -> Sum9/1
  Constant3/1 -> Switch1/1
  sigmaIn/1 -> Switch1/2
  Constant10/1 -> Sum9/2
  Sum9/1 -> sigmaOut/1
  Constant1/1 -> Switch1/3

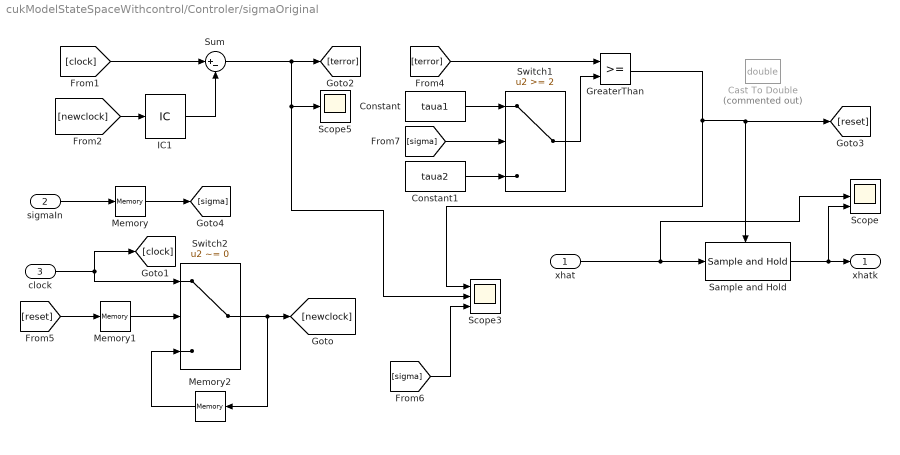
== system cukModelStateSpaceWithcontrol/Controler/sigmaOriginal ==
  xhat : Inport
  sigmaIn : Inport  Port=2
  clock : Inport  Port=3
  Cast To Double : DataTypeConversion  Commented=on  OutDataTypeStr=double
  Constant : Constant  Value=taua1
  Constant1 : Constant  Value=taua2
  GreaterThan : RelationalOperator  OutDataTypeStr=boolean  RndMeth=Simplest
  IC1 : InitialCondition  Value=0
  Memory : Memory  InitialCondition=2  InheritSampleTime=on
  Memory1 : Memory  InitialCondition=2  InheritSampleTime=on
  Memory2 : Memory  InheritSampleTime=on
  Sample and Hold : dspsigops/Sample and Hold  trig=Rising edge  initCond=1  latchinput=off
  Scope : Scope  NumInputPorts=3
  Scope3 : Scope  NumInputPorts=3
  Scope5 : Scope
  Sum : Sum  Inputs=|+-
  Switch1 : Switch  Threshold=2
  Switch2 : Switch  Criteria=u2 ~= 0
  "xhatk " : Outport
  wires:
  xhat/1 -> Scope/2, Sample and Hold/1
  Sample and Hold/1 -> Scope/3, "xhatk "/1
  [clock] -> Sum/1
  Sum/1 -> Scope3/2, Scope5/1, [terror]
  Constant/1 -> Switch1/1
  Constant1/1 -> Switch1/3
  [terror] -> GreaterThan/1
  Switch1/1 -> GreaterThan/2
  GreaterThan/1 -> [reset], Sample and Hold/Trigger, Scope3/1
  clock/1 -> [clock], Switch2/1
  [reset] -> Memory1/1
  Memory1/1 -> Switch2/2
  [newclock] -> IC1/1
  IC1/1 -> Sum/2
  [sigma] -> Scope3/3
  Switch2/1 -> Memory2/1, [newclock]
  Memory2/1 -> Switch2/3
  [sigma] -> Switch1/2
  sigmaIn/1 -> Memory/1
  Memory/1 -> [sigma]

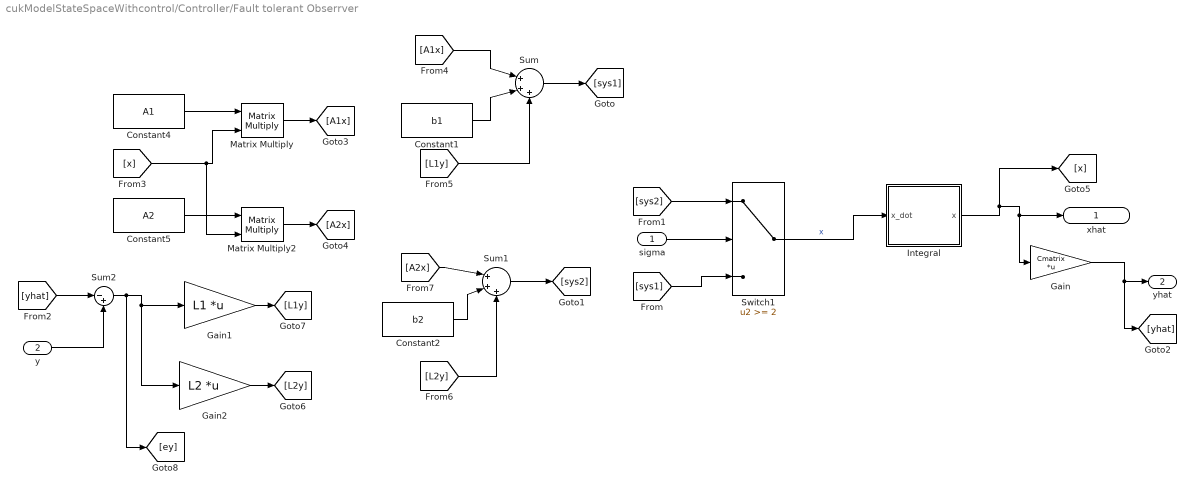
== system cukModelStateSpaceWithcontrol/Controller/Fault tolerant Obserrver ==
  sigma : Inport
  y : Inport  Port=2
  Constant1 : Constant  Value=b1  VectorParams1D=off
  Constant2 : Constant  Value=b2  VectorParams1D=off
  Constant4 : Constant  Value=A1  VectorParams1D=off
  Constant5 : Constant  Value=A2  VectorParams1D=off
  Gain : Gain  Gain=Cmatrix  Multiplication=Matrix(K*u)
  Gain1 : Gain  Gain=L1  Multiplication=Matrix(K*u) (u vector)
  Gain2 : Gain  Gain=L2  Multiplication=Matrix(K*u) (u vector)
  Integral : Subsystem
  Matrix Multiply : Product  Multiplication=Matrix(*)
  Matrix Multiply2 : Product  Multiplication=Matrix(*)
  Sum : Sum  Inputs=|+++
  Sum1 : Sum  Inputs=|+++
  Sum2 : Sum  Inputs=|-+
  Switch1 : Switch  Threshold=2
  xhat : Outport
  yhat : Outport  Port=2
  wires:
  Gain/1 -> [yhat], yhat/1
  Constant1/1 -> Sum/2
  sigma/1 -> Switch1/2
  Matrix Multiply2/1 -> [A2x]
  Sum/1 -> [sys1]
  Constant4/1 -> Matrix Multiply/1
  Constant2/1 -> Sum1/2
  Integral/1(x) -> [x], xhat/1, Gain/1
  Constant5/1 -> Matrix Multiply2/1
  [x] -> Matrix Multiply2/2, Matrix Multiply/2
  Matrix Multiply/1 -> [A1x]
  Sum1/1 -> [sys2]
  [A2x] -> Sum1/1
  [A1x] -> Sum/1
  [L2y] -> Sum1/3
  [yhat] -> Sum2/1
  y/1 -> Sum2/2
  Sum2/1 -> [ey], Gain2/1, Gain1/1
  Gain2/1 -> [L2y]
  Gain1/1 -> [L1y]
  [L1y] -> Sum/3
  [sys2] -> Switch1/1
  [sys1] -> Switch1/3
  Switch1/1 -> Integral/1(x_dot)  "x"

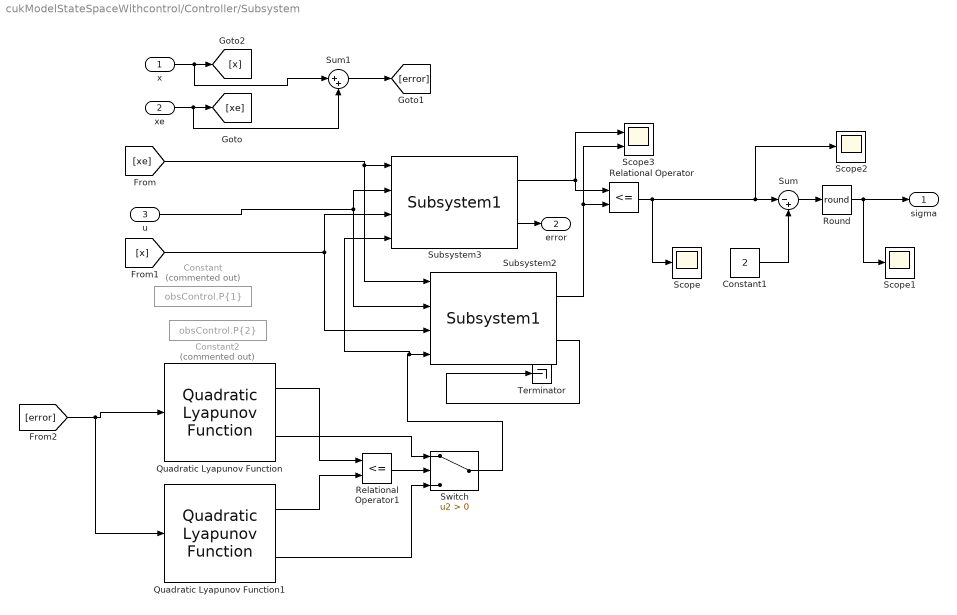
== system cukModelStateSpaceWithcontrol/Controller/Subsystem ==
  x : Inport
  xe : Inport  Port=2
  u : Inport  Port=3
  Constant : Constant  Commented=on  Value=obsControl.P{1}
  Constant1 : Constant  Value=2
  Constant2 : Constant  Commented=on  Value=obsControl.P{2}
  Quadratic Lyapunov Function : PhdLibrary/Quadratic Lyapunov Function  P=P1
      settings: SourceProductName=Phd Diego
  Quadratic Lyapunov Function1 : PhdLibrary/Quadratic Lyapunov Function  P=P2
      settings: SourceProductName=Phd Diego
  Relational Operator : RelationalOperator  Operator=<=  OutDataTypeStr=boolean  RndMeth=Nearest
  Relational Operator1 : RelationalOperator  Operator=<=  OutDataTypeStr=boolean  RndMeth=Nearest
  Round : Rounding  Operator=round
  Scope : Scope
  Scope1 : Scope
  Scope2 : Scope
  Scope3 : Scope  NumInputPorts=2
  Subsystem2 : PhdLibrary/Controllers/Subsystem1  A=A2  B=B2
      settings: SourceProductName=Phd Diego
  Subsystem3 : PhdLibrary/Controllers/Subsystem1  A=A1  B=B1
      settings: SourceProductName=Phd Diego
  Sum : Sum  Inputs=|-+
  Sum1 : Sum  Inputs=|++
  Switch : Switch  Criteria=u2 > Threshold
  Terminator : Terminator
  sigma : Outport
  error : Outport  Port=2
  wires:
  x/1 -> Sum1/1, [x]
  [xe] -> Subsystem2/1, Subsystem3/1
  [x] -> Subsystem3/3, Subsystem2/3
  u/1 -> Subsystem3/2, Subsystem2/2
  Subsystem2/2 -> Terminator/1
  Subsystem3/2 -> error/1
  Subsystem2/1 -> Scope3/2, Relational Operator/2
  Subsystem3/1 -> Relational Operator/1, Scope3/1
  Relational Operator/1 -> Scope2/1, Sum/1, Scope/1
  Constant1/1 -> Sum/2
  Sum/1 -> Round/1
  Round/1 -> Scope1/1, sigma/1
  xe/1 -> [xe], Sum1/2
  Sum1/1 -> [error]
  [error] -> Quadratic Lyapunov Function1/1, Quadratic Lyapunov Function/1
  Quadratic Lyapunov Function1/1 -> Relational Operator1/2
  Relational Operator1/1 -> Switch/2
  Quadratic Lyapunov Function1/2 -> Switch/3
  Quadratic Lyapunov Function/1 -> Relational Operator1/1
  Quadratic Lyapunov Function/2 -> Switch/1
  Switch/1 -> Subsystem3/4, Subsystem2/4

== system cukModelStateSpaceWithcontrol/Controller/Subsystem1 ==
  xhat : Inport
  sigmaIn : Inport  Port=2
  Constant : Constant  Value=0.5
  Constant1 : Constant  Commented=on  Value=0.5
  Memory : Memory  Commented=on
  PWM Generator (DC-DC) : powerlib_meascontrol/Pulse & Signal Generators/PWM Generator (DC-DC)  Fsw=10000  Ts=5e-6
  PWM Generator (DC-DC)1 : powerlib_meascontrol/Pulse & Signal Generators/PWM Generator (DC-DC)  Commented=on  Fsw=10000  Ts=5e-6
  Sample and Hold : dspsigops/Sample and Hold  trig=Either edge  initCond=1  latchinput=off
  Switch : Switch  Commented=on  Threshold=2
  "xhatk " : Outport
  wires:
  xhat/1 -> Sample and Hold/1
  Sample and Hold/1 -> "xhatk "/1
  Constant/1 -> PWM Generator (DC-DC)/1
  sigmaIn/1 -> Memory/1
  Constant1/1 -> PWM Generator (DC-DC)1/1
  PWM Generator (DC-DC)1/1 -> Switch/3
  Memory/1 -> Switch/2
  PWM Generator (DC-DC)/1 -> Sample and Hold/Trigger

== system cukModelStateSpaceWithcontrol/Controller/sigma2PWM ==
  sigmaIn : Inport
  Constant1 : Constant
  Constant10 : Constant  Value=2
  Constant3 : Constant  Value=0
  PWM Generator (DC-DC) : powerlib_meascontrol/Pulse & Signal Generators/PWM Generator (DC-DC)  Fsw=1  Ts=5e-6
  Sum9 : Sum  Inputs=|-+
  Switch1 : Switch  Threshold=2
  sigmaOut : Outport
  wires:
  Switch1/1 -> PWM Generator (DC-DC)/1
  PWM Generator (DC-DC)/1 -> Sum9/1
  Constant3/1 -> Switch1/1
  sigmaIn/1 -> Switch1/2
  Constant10/1 -> Sum9/2
  Sum9/1 -> sigmaOut/1
  Constant1/1 -> Switch1/3

== system cukModelStateSpaceWithcontrol/Observer 2 slidng mode/Integral ==
  x_dot : Inport
  Ground : Ground
  IC : InitialCondition  Value=[x0]
  Integrator1 : Integrator  InitialConditionSource=external  InitialCondition=[-x_e; 0; 0]
  Mux : Mux
  x : Outport
  wires:
  x_dot/1 -> Integrator1/1
  Integrator1/1 -> x/1
  IC/1 -> Integrator1/2
  Mux/1 -> IC/1
  Ground/1 -> Mux/4, Mux/3, Mux/2, Mux/1

== system cukModelStateSpaceWithcontrol/Offset Faults/Fault1 ==
  Constant6 : Constant  Value=0
  Fault 1 : Step  Time=t_f  SampleTime=0
  Sinusoidal : SignalGenerator  Amplitude=fbound  Frequency=f_freq_Hz  Units=rad/sec
  Switch : Switch  Criteria=u2 > Threshold
  fault : Outport
  wires:
  Switch/1 -> fault/1
  Constant6/1 -> Switch/3
  Fault 1/1 -> Switch/2
  Sinusoidal/1 -> Switch/1

== system cukModelStateSpaceWithcontrol/Offset Faults/Fault2 ==
  Constant6 : Constant  Value=0
  Fault 1 : Step  Time=t_f  SampleTime=0
  Sinusoidal : SignalGenerator  Amplitude=fbound  Frequency=f_freq_Hz  Units=rad/sec
  Switch : Switch  Criteria=u2 > Threshold
  fault : Outport
  wires:
  Switch/1 -> fault/1
  Constant6/1 -> Switch/3
  Fault 1/1 -> Switch/2
  Sinusoidal/1 -> Switch/1

== system cukModelStateSpaceWithcontrol/Offset Faults/Fault4 ==
  Constant6 : Constant  Value=0
  Fault 1 : Step  Time=t_f  SampleTime=0
  Sinusoidal : SignalGenerator  Amplitude=fbound  Frequency=f_freq_Hz  Units=rad/sec
  Switch : Switch  Criteria=u2 > Threshold
  fault : Outport
  wires:
  Switch/1 -> fault/1
  Constant6/1 -> Switch/3
  Fault 1/1 -> Switch/2
  Sinusoidal/1 -> Switch/1

== system cukModelStateSpaceWithcontrol/Subsystem2/Subsystem ==
  f(t) : Inport
  Constant : Constant  Value=M1
  Constant3 : Constant  Value=M2
  Gain1 : Gain  Gain=N1
  Gain2 : Gain  Gain=N2
  Matrix Multiply1 : Product  Multiplication=Matrix(*)
  Matrix Multiply3 : Product  Multiplication=Matrix(*)
  delta1 : Outport
  delta2 : Outport  Port=2
  wires:
  f(t)/1 -> Gain1/1, Gain2/1
  Constant3/1 -> Matrix Multiply1/1
  Gain1/1 -> Matrix Multiply3/2
  Constant/1 -> Matrix Multiply3/1
  Gain2/1 -> Matrix Multiply1/2
  Matrix Multiply3/1 -> delta1/1
  Matrix Multiply1/1 -> delta2/1

== system cukModelStateSpaceWithcontrol/Subsystem2/Subsystem1 ==
  Step1 : Step  Time=0.025  SampleTime=0
  Step10 : Step  Time=0.25  After=-1  SampleTime=0
  Step2 : Step  Time=0.05  After=-1  SampleTime=0
  Step3 : Step  Time=0.075  After=-1  SampleTime=0
  Step4 : Step  Time=0.1  SampleTime=0
  Step5 : Step  Time=0.125  SampleTime=0
  Step6 : Step  Time=0.15  After=-1  SampleTime=0
  Step7 : Step  Time=0.175  After=-1  SampleTime=0
  Step8 : Step  Time=0.2  SampleTime=0
  Step9 : Step  Time=0.225  SampleTime=0
  Sum{,1..8} (9 alike) : Sum  Inputs=|++
  SquareUncertainty : Outport
  wires:
  Step1/1 -> Sum/1
  Step2/1 -> Sum/2
  Step4/1 -> Sum1/2
  Step3/1 -> Sum1/1
  Sum/1 -> Sum2/1
  Step7/1 -> Sum4/1
  Step6/1 -> Sum3/2
  Step8/1 -> Sum4/2
  Sum4/1 -> Sum7/2
  Step5/1 -> Sum3/1
  Sum3/1 -> Sum7/1
  Sum1/1 -> Sum2/2
  Step9/1 -> Sum5/1
  Step10/1 -> Sum5/2
  Sum5/1 -> Sum8/2
  Sum7/1 -> Sum8/1
  Sum2/1 -> Sum6/1
  Sum8/1 -> Sum6/2
  Sum6/1 -> SquareUncertainty/1  "squareUncertainty"

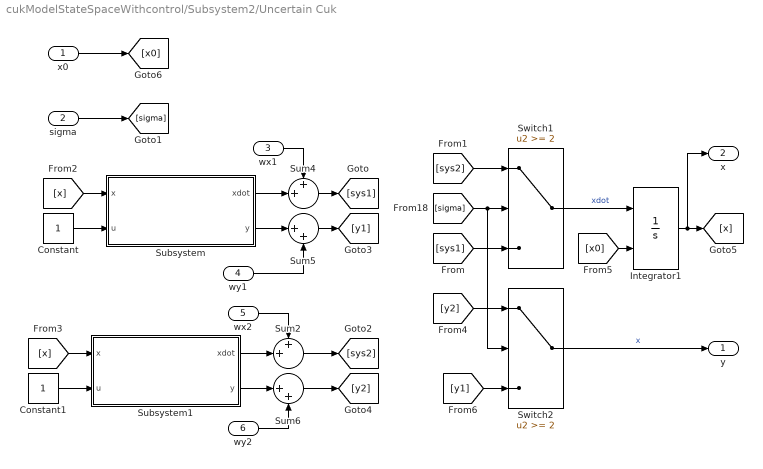
== system cukModelStateSpaceWithcontrol/Subsystem2/Uncertain Cuk ==
  x0 : Inport
  sigma : Inport  Port=2
  wx1 : Inport  Port=3
  wy1 : Inport  Port=4
  wx2 : Inport  Port=5
  wy2 : Inport  Port=6
  Constant : Constant
  Constant1 : Constant
  Integrator1 : Integrator  InitialConditionSource=external  InitialCondition=[-x_e; 0; 0]
  Subsystem : Subsystem  mask{A=A1, B=B1, C=C1}
      mask prompts: A "Matrix A"; B "Matrix B"; C "Matrix C"
      mask Display: disp('Static State Space \n xdot = Ax+Bu\n y =Cx')
  Subsystem1 : Subsystem  mask{A=A2, B=B2, C=C2}
      mask prompts: A "Matrix A"; B "Matrix B"; C "Matrix C"
      mask Display: disp('Static State Space \n xdot = Ax+Bu\n y =Cx')
  Sum2 : Sum  Inputs=++|
  Sum4 : Sum  Inputs=++|
  Sum5 : Sum  Inputs=|++
  Sum6 : Sum  Inputs=|++
  Switch1 : Switch  Threshold=2
  Switch2 : Switch  Threshold=2
  y : Outport
  x : Outport  Port=2
  wires:
  [sys2] -> Switch1/1
  [sys1] -> Switch1/3
  [sigma] -> Switch2/2, Switch1/2
  Subsystem/1(xdot) -> Sum4/2
  Subsystem/2(y) -> Sum5/1
  Sum4/1 -> [sys1]
  Sum5/1 -> [y1]
  [x] -> Subsystem/1(x)
  Constant/1 -> Subsystem/2(u)
  Switch1/1 -> Integrator1/1  "xdot"
  [x0] -> Integrator1/2
  Integrator1/1 -> x/1, [x]
  Sum6/1 -> [y2]
  Sum2/1 -> [sys2]
  Subsystem1/2(y) -> Sum6/1
  [x] -> Subsystem1/1(x)
  Subsystem1/1(xdot) -> Sum2/2
  Constant1/1 -> Subsystem1/2(u)
  [y2] -> Switch2/1
  [y1] -> Switch2/3
  Switch2/1 -> y/1  "x"
  sigma/1 -> [sigma]
  x0/1 -> [x0]
  wx1/1 -> Sum4/1
  wy1/1 -> Sum5/2
  wx2/1 -> Sum2/1
  wy2/1 -> Sum6/2

== system cukModelStateSpaceWithcontrol/Subsystem2/Uncertainties ==
  note: DeltaAx
  note: DeltaBu
  note: DeltaCx
  x : Inport
  u : Inport  Port=2
  delta(t) : Inport  Port=3
  Subsystem1 : Subsystem  mask{M=Mbsigma{1}, N=Nbsigma{1}}
      mask prompts: M "M matrix"; N "N matrix"
      mask DialogControl DescTextVar Prompt: Uncertainties matrices of type \DeltaA = delta(t)*MaNa*x(t)
      mask Display: disp('Norm-bounded \n uncertainty')
  Subsystem2 : Subsystem  mask{M=Mbsigma{2}, N=Nbsigma{2}}
      mask prompts: M "M matrix"; N "N matrix"
      mask DialogControl DescTextVar Prompt: Uncertainties matrices of type \DeltaA = delta(t)*MaNa*x(t)
      mask Display: disp('Norm-bounded \n uncertainty')
  Subsystem3 : Subsystem  mask{M=Masigma{1}, N=Nasigma{1}}
      mask prompts: M "M matrix"; N "N matrix"
      mask DialogControl DescTextVar Prompt: Uncertainties matrices of type \DeltaA = delta(t)*MaNa*x(t)
      mask Display: disp('Norm-bounded \n uncertainty')
  Subsystem4 : Subsystem  mask{M=Masigma{2}, N=Nasigma{2}}
      mask prompts: M "M matrix"; N "N matrix"
      mask DialogControl DescTextVar Prompt: Uncertainties matrices of type \DeltaA = delta(t)*MaNa*x(t)
      mask Display: disp('Norm-bounded \n uncertainty')
  Subsystem7 : Subsystem  mask{M=Mcsigma{1}, N=Ncsigma{1}}
      mask prompts: M "M matrix"; N "N matrix"
      mask DialogControl DescTextVar Prompt: Uncertainties matrices of type \DeltaA = delta(t)*MaNa*x(t)
      mask Display: disp('Norm-bounded \n uncertainty')
  Subsystem8 : Subsystem  mask{M=Mcsigma{2}, N=Ncsigma{2}}
      mask prompts: M "M matrix"; N "N matrix"
      mask DialogControl DescTextVar Prompt: Uncertainties matrices of type \DeltaA = delta(t)*MaNa*x(t)
      mask Display: disp('Norm-bounded \n uncertainty')
  DeltaA1x : Outport
  DeltaA2x : Outport  Port=2
  DeltaB1u : Outport  Port=3
  DeltaB2u : Outport  Port=4
  DeltaC1x : Outport  Port=5
  DeltaC2x : Outport  Port=6
  wires:
  u/1 -> [u]
  Subsystem3/1(DeltaAx) -> DeltaA1x/1
  Subsystem4/1(DeltaAx) -> DeltaA2x/1
  x/1 -> [x]
  delta(t)/1 -> [delta]
  [delta] -> Subsystem3/1(delta(t)), Subsystem4/1(delta(t))
  [x] -> Subsystem4/2(x), Subsystem3/2(x)
  Subsystem2/1(DeltaAx) -> DeltaB2u/1
  [delta] -> Subsystem1/1(delta(t)), Subsystem2/1(delta(t))
  Subsystem1/1(DeltaAx) -> DeltaB1u/1
  [u] -> Subsystem2/2(x), Subsystem1/2(x)
  Subsystem8/1(DeltaAx) -> DeltaC2x/1
  Subsystem7/1(DeltaAx) -> DeltaC1x/1
  [delta] -> Subsystem7/1(delta(t)), Subsystem8/1(delta(t))
  [x] -> Subsystem8/2(x), Subsystem7/2(x)

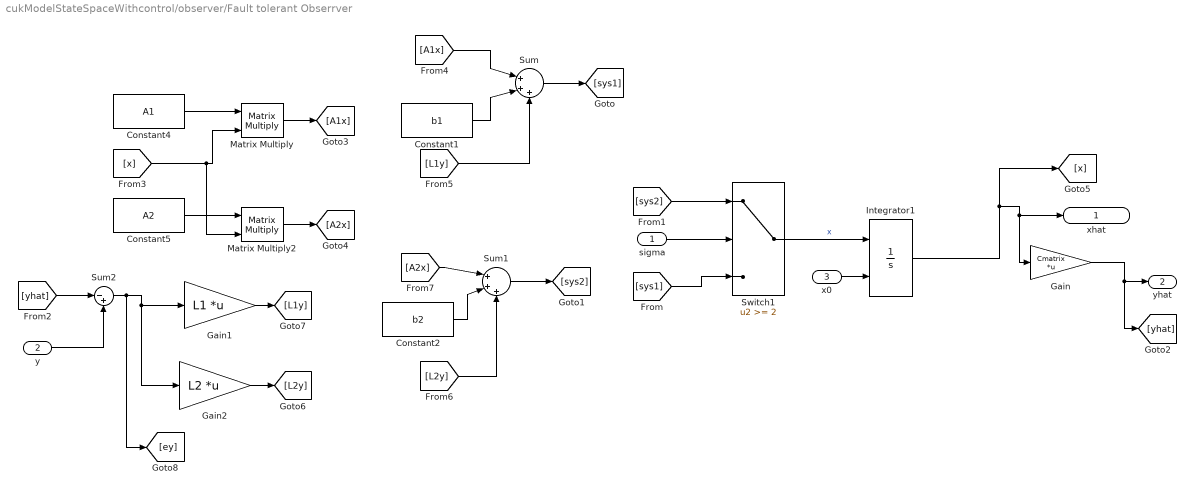
== system cukModelStateSpaceWithcontrol/observer/Fault tolerant Obserrver ==
  sigma : Inport
  y : Inport  Port=2
  x0 : Inport  Port=3
  Constant1 : Constant  Value=b1  VectorParams1D=off
  Constant2 : Constant  Value=b2  VectorParams1D=off
  Constant4 : Constant  Value=A1  VectorParams1D=off
  Constant5 : Constant  Value=A2  VectorParams1D=off
  Gain : Gain  Gain=Cmatrix  Multiplication=Matrix(K*u)
  Gain1 : Gain  Gain=L1  Multiplication=Matrix(K*u) (u vector)
  Gain2 : Gain  Gain=L2  Multiplication=Matrix(K*u) (u vector)
  Integrator1 : Integrator  InitialConditionSource=external  InitialCondition=[-x_e; 0; 0]
  Matrix Multiply : Product  Multiplication=Matrix(*)
  Matrix Multiply2 : Product  Multiplication=Matrix(*)
  Sum : Sum  Inputs=|+++
  Sum1 : Sum  Inputs=|+++
  Sum2 : Sum  Inputs=|-+
  Switch1 : Switch  Threshold=2
  xhat : Outport
  yhat : Outport  Port=2
  wires:
  Gain/1 -> [yhat], yhat/1
  Constant1/1 -> Sum/2
  sigma/1 -> Switch1/2
  Matrix Multiply2/1 -> [A2x]
  Sum/1 -> [sys1]
  Constant4/1 -> Matrix Multiply/1
  Constant2/1 -> Sum1/2
  Integrator1/1 -> [x], xhat/1, Gain/1
  Constant5/1 -> Matrix Multiply2/1
  [x] -> Matrix Multiply2/2, Matrix Multiply/2
  Matrix Multiply/1 -> [A1x]
  Sum1/1 -> [sys2]
  [A2x] -> Sum1/1
  [A1x] -> Sum/1
  [L2y] -> Sum1/3
  [yhat] -> Sum2/1
  y/1 -> Sum2/2
  Sum2/1 -> [ey], Gain2/1, Gain1/1
  Gain2/1 -> [L2y]
  Gain1/1 -> [L1y]
  [L1y] -> Sum/3
  [sys2] -> Switch1/1
  [sys1] -> Switch1/3
  x0/1 -> Integrator1/2
  Switch1/1 -> Integrator1/1  "x"

== system cukModelStateSpaceWithcontrol/Controller/Fault tolerant Obserrver/Integral ==
  x_dot : Inport
  Ground : Ground
  IC : InitialCondition  Value=[x0]
  Integrator1 : Integrator  InitialConditionSource=external  InitialCondition=[-x_e; 0; 0]
  Mux : Mux
  x : Outport
  wires:
  x_dot/1 -> Integrator1/1
  Integrator1/1 -> x/1
  IC/1 -> Integrator1/2
  Mux/1 -> IC/1
  Ground/1 -> Mux/4, Mux/3, Mux/2, Mux/1

== system cukModelStateSpaceWithcontrol/Subsystem2/Uncertain Cuk/Subsystem ==
  x : Inport
  u : Inport  Port=2
  Gain : Gain  Gain=B  Multiplication=Matrix(K*u) (u vector)
  Gain1 : Gain  Gain=A  Multiplication=Matrix(K*u) (u vector)
  Gain2 : Gain  Gain=C  Multiplication=Matrix(K*u) (u vector)
  Sum : Sum  Inputs=|++
  xdot : Outport
  y : Outport  Port=2
  wires:
  u/1 -> Gain/1
  x/1 -> Gain2/1, Gain1/1
  Gain1/1 -> Sum/1
  Gain/1 -> Sum/2
  Sum/1 -> xdot/1
  Gain2/1 -> y/1

== system cukModelStateSpaceWithcontrol/Subsystem2/Uncertain Cuk/Subsystem1 ==
  x : Inport
  u : Inport  Port=2
  Gain : Gain  Gain=B  Multiplication=Matrix(K*u) (u vector)
  Gain1 : Gain  Gain=A  Multiplication=Matrix(K*u) (u vector)
  Gain2 : Gain  Gain=C  Multiplication=Matrix(K*u) (u vector)
  Sum : Sum  Inputs=|++
  xdot : Outport
  y : Outport  Port=2
  wires:
  u/1 -> Gain/1
  x/1 -> Gain2/1, Gain1/1
  Gain1/1 -> Sum/1
  Gain/1 -> Sum/2
  Sum/1 -> xdot/1
  Gain2/1 -> y/1

== system cukModelStateSpaceWithcontrol/Subsystem2/Uncertainties/Subsystem1 ==
  delta(t) : Inport
  x : Inport  Port=2
  Constant : Constant  Value=M
  Constant1 : Constant  Value=N
  Matrix Multiply1 : Product
  Matrix Multiply2 : Product  Multiplication=Matrix(*)
  Matrix Multiply3 : Product  Multiplication=Matrix(*)
  DeltaAx : Outport
  wires:
  Constant/1 -> Matrix Multiply3/1
  Constant1/1 -> Matrix Multiply3/2
  Matrix Multiply3/1 -> Matrix Multiply1/2
  delta(t)/1 -> Matrix Multiply1/1
  Matrix Multiply1/1 -> Matrix Multiply2/1
  x/1 -> Matrix Multiply2/2
  Matrix Multiply2/1 -> DeltaAx/1

== system cukModelStateSpaceWithcontrol/Subsystem2/Uncertainties/Subsystem2 ==
  delta(t) : Inport
  x : Inport  Port=2
  Constant : Constant  Value=M
  Constant1 : Constant  Value=N
  Matrix Multiply1 : Product
  Matrix Multiply2 : Product  Multiplication=Matrix(*)
  Matrix Multiply3 : Product  Multiplication=Matrix(*)
  DeltaAx : Outport
  wires:
  Constant/1 -> Matrix Multiply3/1
  Constant1/1 -> Matrix Multiply3/2
  Matrix Multiply3/1 -> Matrix Multiply1/2
  delta(t)/1 -> Matrix Multiply1/1
  Matrix Multiply1/1 -> Matrix Multiply2/1
  x/1 -> Matrix Multiply2/2
  Matrix Multiply2/1 -> DeltaAx/1

== system cukModelStateSpaceWithcontrol/Subsystem2/Uncertainties/Subsystem3 ==
  delta(t) : Inport
  x : Inport  Port=2
  Constant : Constant  Value=M
  Constant1 : Constant  Value=N
  Matrix Multiply1 : Product
  Matrix Multiply2 : Product  Multiplication=Matrix(*)
  Matrix Multiply3 : Product  Multiplication=Matrix(*)
  DeltaAx : Outport
  wires:
  Constant/1 -> Matrix Multiply3/1
  Constant1/1 -> Matrix Multiply3/2
  Matrix Multiply3/1 -> Matrix Multiply1/2
  delta(t)/1 -> Matrix Multiply1/1
  Matrix Multiply1/1 -> Matrix Multiply2/1
  x/1 -> Matrix Multiply2/2
  Matrix Multiply2/1 -> DeltaAx/1

== system cukModelStateSpaceWithcontrol/Subsystem2/Uncertainties/Subsystem4 ==
  delta(t) : Inport
  x : Inport  Port=2
  Constant : Constant  Value=M
  Constant1 : Constant  Value=N
  Matrix Multiply1 : Product
  Matrix Multiply2 : Product  Multiplication=Matrix(*)
  Matrix Multiply3 : Product  Multiplication=Matrix(*)
  DeltaAx : Outport
  wires:
  Constant/1 -> Matrix Multiply3/1
  Constant1/1 -> Matrix Multiply3/2
  Matrix Multiply3/1 -> Matrix Multiply1/2
  delta(t)/1 -> Matrix Multiply1/1
  Matrix Multiply1/1 -> Matrix Multiply2/1
  x/1 -> Matrix Multiply2/2
  Matrix Multiply2/1 -> DeltaAx/1

== system cukModelStateSpaceWithcontrol/Subsystem2/Uncertainties/Subsystem7 ==
  delta(t) : Inport
  x : Inport  Port=2
  Constant : Constant  Value=M
  Constant1 : Constant  Value=N
  Matrix Multiply1 : Product
  Matrix Multiply2 : Product  Multiplication=Matrix(*)
  Matrix Multiply3 : Product  Multiplication=Matrix(*)
  DeltaAx : Outport
  wires:
  Constant/1 -> Matrix Multiply3/1
  Constant1/1 -> Matrix Multiply3/2
  Matrix Multiply3/1 -> Matrix Multiply1/2
  delta(t)/1 -> Matrix Multiply1/1
  Matrix Multiply1/1 -> Matrix Multiply2/1
  x/1 -> Matrix Multiply2/2
  Matrix Multiply2/1 -> DeltaAx/1

== system cukModelStateSpaceWithcontrol/Subsystem2/Uncertainties/Subsystem8 ==
  delta(t) : Inport
  x : Inport  Port=2
  Constant : Constant  Value=M
  Constant1 : Constant  Value=N
  Matrix Multiply1 : Product
  Matrix Multiply2 : Product  Multiplication=Matrix(*)
  Matrix Multiply3 : Product  Multiplication=Matrix(*)
  DeltaAx : Outport
  wires:
  Constant/1 -> Matrix Multiply3/1
  Constant1/1 -> Matrix Multiply3/2
  Matrix Multiply3/1 -> Matrix Multiply1/2
  delta(t)/1 -> Matrix Multiply1/1
  Matrix Multiply1/1 -> Matrix Multiply2/1
  x/1 -> Matrix Multiply2/2
  Matrix Multiply2/1 -> DeltaAx/1
